simulink model "Task3_MaximumPowerPointTracking"  (R2025b)
settings: Solver=VariableStepAuto  StartTime=0.0  StopTime=100  RelTol=1e-3
undefined symbols (not defined in the file): Ts
libraries: fl_lib x6, nesl_utility x6, ee_lib x2
settings Model: Creator=gdudgeon  LastModifiedBy=Tiziano
settings RTWCC: GPUComputeCapability=3.5

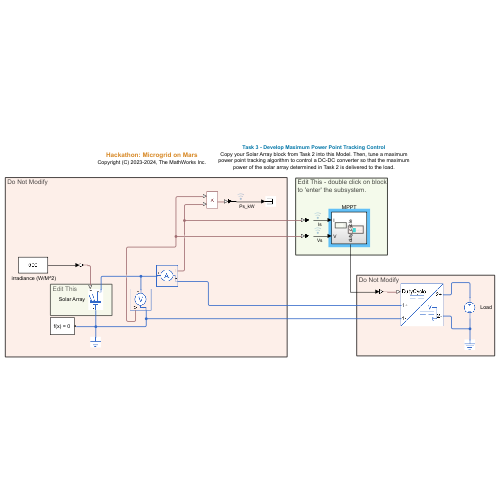
[thumbnail: Simulink's stored preview of the top-level diagram]
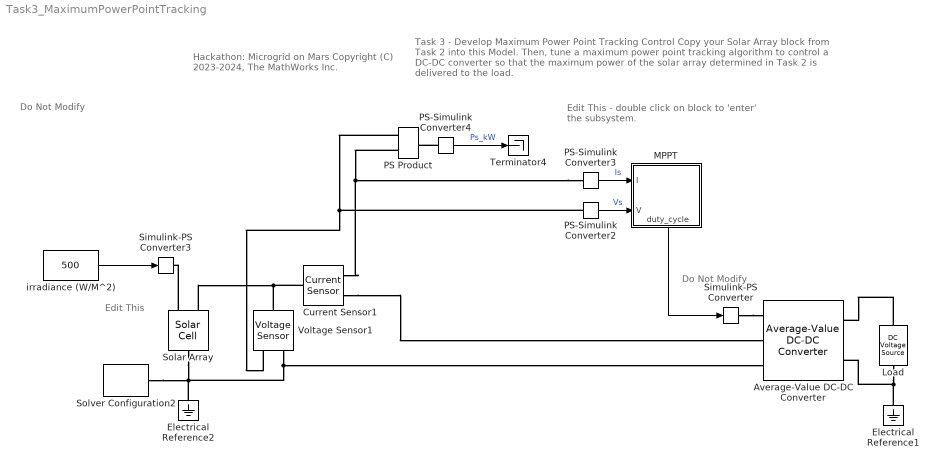
== system Task3_MaximumPowerPointTracking ==
  note: Edit This
  note: Do Not Modify
  note: Edit This - double click on block
      | to 'enter' the subsystem.
  note: Do Not Modify
  note: Task 3 - Develop Maximum Power Point Tracking Control
      | Copy your Solar Array block from Task 2 into this Model. Then, tune a maximum power point tracking algorithm to control a DC-DC converter so that the maximum power of the solar array determined in Task 2 is delivered to the load.
  note: Hackathon: Microgrid on Mars
      | Copyright (C) 2023-2024, The MathWorks Inc.
  " irradiance (W/M^2)" : Constant  Value=500
  Average-Value DC-DC Converter : ee_lib/Semiconductors & Converters/Converters/Average-Value DC-DC Converter  implementation_option=ee.enum.converters.implementation.behavioral  converter_type=ee.enum.converters.dcdctype.buckboost  control_option=ee.enum.converters.controlinput.dutycycle  efficiency_option=ee.enum.converters.efficiency.constant  efficiency_fixed=100  i_vec=[0, 2, 5] A  efficiency_vec=[90, 95, 98]  Lf=1e-6 H  Rl=0 Ohm  Cf=1e-7 F  Rc=1e-6 Ohm  iL_specify=off  iL_priority=High  iL=0 A  iL_nominal_specify=off  iL_nominal_value=1  iL_nominal_unit=A  vc_specify=off  vc_priority=High  vc=0 V  vc_nominal_specify=off  vc_nominal_value=1  vc_nominal_unit=V
      settings: InternalSimscapePortConfiguration="{\"Bottom\":[],\"Left\":[{\"id\":\"DutyCycle\",\"label\":\"DutyCycle\",\"type\":\"input\"},{\"id\":\"p1\",\"label\":\"1+\",\"type\":\"foundation.electrical.electrical\"},{\"id\":\"n1\",\"label\":\"1-\",\"type\":\"foundation.electrical.electrical\"}],\"Right\":[{\"id\":\"p2\",\"label\":\"2+\",\"type\":\"foundation.electrical.electrical\"},{\"id\":\"n2\",\"label\":\"2-\",\"type\":\"foundation.electrical.electrical\"}],\"Top\":[]}"
  Current Sensor1 : fl_lib/Electrical/Electrical Sensors/Current Sensor
  Electrical Reference1 : fl_lib/Electrical/Electrical Elements/Electrical Reference
  Electrical Reference2 : fl_lib/Electrical/Electrical Elements/Electrical Reference
  Load : fl_lib/Electrical/Electrical Sources/DC Voltage Source  v0=500 V
  MPPT : Subsystem
      settings: PortSchema="{\"entries\":[{\"content\":{\"sides\":[{\"content\":{\"connectorIds\":[\"In1\",\"In2\"]},\"type\":\"ConnectorPlacement.EquallySpacedRectSide\",\"uuid\":\"1516a238-5333-4be9-a665-0b0f3b54c673\"},{\"content\":{\"side\":\"RIGHT\"},\"type\":\"ConnectorPlacement.EquallySpacedRectSide\",\"uuid\":\"a9b904e5-6957-4e5e-80be-9121abf01a93\"},{\"content\":{\"side\":\"TOP\"},\"type\":\"ConnectorPlacement.EquallySpacedRectSide\",\"uuid\":\"2fbf786c-21bd-4a0b-9993-3a26cd9abc14\"},{\"content\":{\"connectorIds\":[\"Out1\"],\"side\":\"BOTTOM\"},\"type\":\"ConnectorPlacement.EquallySpacedRectSide\",\"uuid\":\"4a6852c2-3e94-4c8b-bb3b-3edfe1e23dcf\"}]},\"type\":\"ConnectorPlacement.EquallySpacedConnector\",\"uuid\":\"28e82bcc-054b-4eaa-b165-f34ac33aacb4\"}],\"packageUris\":[\"http://schema.mathworks.com/mf0/Connector/R2020b\"],\"version\":\"1.0\"}"
  PS Product : fl_lib/Physical Signals/Functions/PS Product
  PS-Simulink Converter2 : nesl_utility/PS-Simulink Converter  PhysicalDomain=network_engine_domain  SubClassName=ps_output  LeftPortType=input  RightPortType=output  PseudoPeriodic=off  Frequencies=[]  VectorFormat=inherit  Unit=inherit  AffineConversion=off
  PS-Simulink Converter3 : nesl_utility/PS-Simulink Converter  PhysicalDomain=network_engine_domain  SubClassName=ps_output  LeftPortType=input  RightPortType=output  PseudoPeriodic=off  Frequencies=[]  VectorFormat=inherit  Unit=inherit  AffineConversion=off
  PS-Simulink Converter4 : nesl_utility/PS-Simulink Converter  PhysicalDomain=network_engine_domain  SubClassName=ps_output  LeftPortType=input  RightPortType=output  PseudoPeriodic=off  Frequencies=[]  VectorFormat=inherit  Unit=kW  AffineConversion=off
  Simulink-PS Converter : nesl_utility/Simulink-PS Converter  PhysicalDomain=network_engine_domain  SubClassName=ps_input  LeftPortType=input  RightPortType=output  PseudoPeriodic=off  Frequencies=[]  NoiseDistribution=none  NoiseParameters=[]  Unit=1  AffineConversion=off  FilteringAndDerivatives=provide  SimscapeFilterOrder=1  InputFilterTimeConstant=0.001  UdotUserProvided=0
  Simulink-PS Converter3 : nesl_utility/Simulink-PS Converter  PhysicalDomain=network_engine_domain  SubClassName=ps_input  LeftPortType=input  RightPortType=output  PseudoPeriodic=off  Frequencies=[]  NoiseDistribution=none  NoiseParameters=[]  Unit=W/m^2  AffineConversion=off  FilteringAndDerivatives=provide  SimscapeFilterOrder=1  InputFilterTimeConstant=0.001  UdotUserProvided=0
  Solar Array : ee_lib/Sources/Solar Cell  prm=1  Isc=10.6 A  Voc=0.61 V  Is=1e-6 A  Is2=0 A  Iph=7.34 A  Ir0=500 W/m^2  ec=1.5  N2=2  Rs=0 Ohm  Rp=inf Ohm  N_series=1000  N_parallel=10  TIPH1=0 1/K  EG=1.11 eV  TXIS1=3  TXIS2=3  TRS1=0  TRP1=0  Tmeas=25 degC  TFIXED=25 degC  thermal_mass=100 J/K  initial_temperature=25 degC
  Solver Configuration2 : nesl_utility/Solver Configuration  PhysicalDomain=network_engine_domain  SubClassName=solver  LeftPortType=input  RightPortType=generic  Tones=[]  Harmonics=[]  SimulateNoise=off  Profile=off  UseLocalSampling=off  EnableSwitchedLinearOptims=on  FrequencyDomain=off  UseCCode=off  RelTol=0.001  AbsTol=0.001  MinStep=1e-09  ToWorkspace=off  RevertToSquareIcSolve=off  NumHomotopyIterations=100  PhasorMode=off  PhasorModeNumHarmonics=1  ConsistencySolver=NEWTON_XTOL_AFTER_FTOL  IndexReductionMethod=None  DoDC=off  ResidualTolerance=1e-09  ConsistencyTolSource=GLOBAL  ConsistencyAbsTol=0.001  ConsistencyRelTol=0.001  ConsistencyTolFactor=0.001  UseLocalSolver=on  LocalSolverChoice=NE_BACKWARD_EULER_ADVANCER  ResolveIndetEquations=off  FunctionEvalNumThread=1  LocalSolverSampleTime=Ts  DoFixedCost=on  MaxNonlinIter=1  MaxModeIter=2  ComputeImpulses=off  ImpulseIterations=2  LinearAlgebra=Sparse  LinearAlgebraNumThread=0  EquationFormulation=NE_TIME_EF  DelaysMemoryBudget=1024  AutomaticFiltering=off  FilteringTimeConstant=0.001  PartitionStorageMethod=AS_NEEDED  PartitionMemoryBudget=1024  PartitionMethod=ROBUST  MultibodyUseLocalSolver=off  MultibodyLocalSolverChoice=ODE1  MultibodyLocalSolverSampleTime=0.001
  Terminator4 : Terminator
  Voltage Sensor1 : fl_lib/Electrical/Electrical Sensors/Voltage Sensor
  wires:
  MPPT/1(duty_cycle) -> Simulink-PS Converter/1
  " irradiance (W/M^2)"/1 -> Simulink-PS Converter3/1
  PS-Simulink Converter2/1 -> MPPT/2(V)  "Vs"
  PS-Simulink Converter3/1 -> MPPT/1(I)  "Is"
  PS-Simulink Converter4/1 -> Terminator4/1  "Ps_kW"
  connections:
  Current Sensor1/LConn1 -- Solar Array/LConn2 -- Voltage Sensor1/LConn1
  Average-Value DC-DC Converter/RConn2 -- Load/RConn1 -- Electrical Reference1/LConn1
  PS-Simulink Converter2/LConn1 -- Voltage Sensor1/RConn1 -- PS Product/LConn1
  Solver Configuration2/RConn1 -- Voltage Sensor1/RConn2 -- Average-Value DC-DC Converter/LConn3 -- Solar Array/RConn1 -- Electrical Reference2/LConn1
  PS-Simulink Converter3/LConn1 -- Current Sensor1/RConn1 -- PS Product/LConn2
  PS-Simulink Converter4/LConn1 -- PS Product/RConn1
  Simulink-PS Converter/RConn1 -- Average-Value DC-DC Converter/LConn1
  Current Sensor1/RConn2 -- Average-Value DC-DC Converter/LConn2
  Load/LConn1 -- Average-Value DC-DC Converter/RConn1
  Solar Array/LConn1 -- Simulink-PS Converter3/RConn1

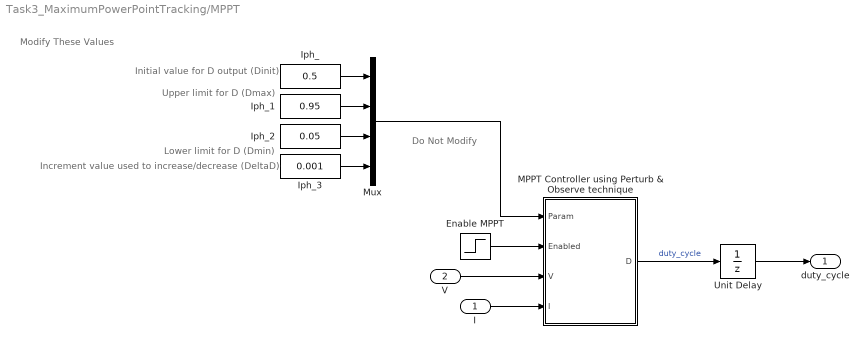
== system Task3_MaximumPowerPointTracking/MPPT ==
  note: Do Not Modify
  note: Modify These Values
  note: Lower limit for D (Dmin)
  note: Upper limit for D (Dmax)
  note: Increment value used to increase/decrease (DeltaD)
  note: Initial value for D output (Dinit)
  I : Inport
  V : Inport  Port=2
  Enable MPPT : Step  Time=0.1  Before=1  SampleTime=0
  Iph_ : Constant  Value=0.5
  Iph_1 : Constant  Value=0.95
  Iph_2 : Constant  Value=0.05
  Iph_3 : Constant  Value=0.001
  "MPPT Controller using Perturb & Observe technique " : MATLAB Function  SystemSampleTime=Ts
  Mux : Mux
  Unit Delay : UnitDelay  InitialCondition=1  SampleTime=-1  HasFrameUpgradeWarning=on
  duty_cycle : Outport
  wires:
  Unit Delay/1 -> duty_cycle/1
  I/1 -> "MPPT Controller using Perturb & Observe technique "/4(I)
  Enable MPPT/1 -> "MPPT Controller using Perturb & Observe technique "/2(Enabled)
  Iph_3/1 -> Mux/4
  "MPPT Controller using Perturb & Observe technique "/1(D) -> Unit Delay/1  "duty_cycle"
  Iph_2/1 -> Mux/3
  Iph_/1 -> Mux/1
  Iph_1/1 -> Mux/2
  Mux/1 -> "MPPT Controller using Perturb & Observe technique "/1(Param)
  V/1 -> "MPPT Controller using Perturb & Observe technique "/3(V)

== matlab function Task3_MaximumPowerPointTracking/MPPT/MPPT Controller using Perturb & Observe technique  ==
  settings: updateMethod=DISCRETE  sampleTime=Ts
  data: Param input; Enabled input; V input; I input; D output
function D  = PandO(Param, Enabled, V, I)

% MPPT controller based on the Perturb & Observe algorithm.

% D output = Duty cycle of the boost converter (value between 0 and 1)
%
% Enabled input = 1 to enable the MPPT controller
% V input = PV array terminal voltage (V)
% I input = PV array current (A)
%
% Param input:
Dinit = Param(1);  %Initial value for D output
Dmax = Param(2);   %Maximum value for D
Dmin = Param(3);   %Minimum value for D
deltaD = Param(4); %Increment value used to increase/decrease the duty cycle D
% ( increasing D = decreasing Vref )
%  

persistent Vold Pold Dold;


if isempty(Vold)
    Vold=0;
    Pold=0;
    Dold=Dinit;
end

P= V*I;
dV= V - Vold;
dP= P - Pold;

 if dP ~= 0 && Enabled ~=0
     if dP < 0
         if dV < 0
             D = Dold - deltaD;
         else
             D = Dold + deltaD;
         end
     else
         if dV < 0
             D = Dold + deltaD;
         else
             D = Dold - deltaD;  
         end    
     end
 else D = Dold;
 end

if D >= Dmax || D<= Dmin
    D=Dold;
end

Dold=D;
Vold=V;
Pold=P;
